simulink model "part4model"  (R2019b)
settings: Solver=VariableStepAuto  StartTime=0.0  StopTime=10.0  RelTol=1e-3
values from neighbouring files (symbols this model uses):
  encGain = (2*pi)/4096    (= 0.00153398078789)    [DC_Motor_Analysis.m]    (also in Part2.m; Part3.m; lqrPoles.mat; robust.mat)
  K_lqr = K_tilde(1:2)    [DC_Motor_Analysis.m]    (also in Part4.m = K(1:2); lqrPoles.mat = [-0.852723665026 -39.4121845033])
  ka = K(end)    [Part3.m]    (also in Part4.m; lqrPoles.mat = 316.227766017)
settings Model: Creator=justinf  LastModifiedBy=justinf

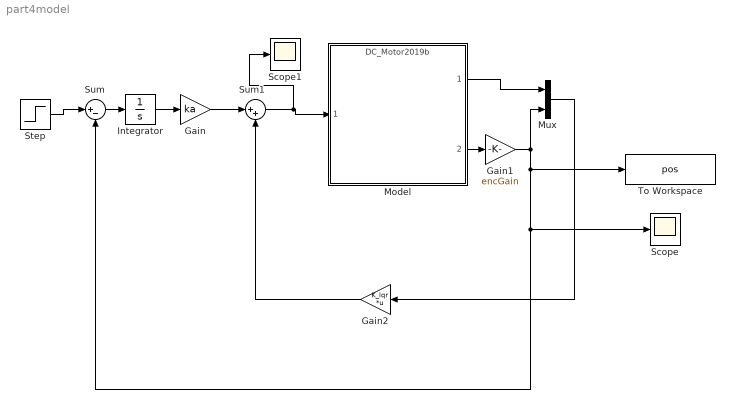
== system part4model ==
  Gain : Gain  Gain=ka
  Gain1 : Gain  Gain=encGain
  Gain2 : Gain  Gain=K_lqr  Multiplication=Matrix(K*u)
  Integrator : Integrator
  Model : ModelReference  ModelNameDialog=DC_Motor2019b.slxp  ModelReferenceVersion=1.20  CopyOfModelProtected=on
  Mux : Mux  Inputs=2
  Scope : Scope
  Scope1 : Scope
  Step : Step  Time=0  SampleTime=0
  Sum : Sum  Inputs=|+-
  Sum1 : Sum  Inputs=|++
  To Workspace : ToWorkspace  VariableName=pos  SampleTime=-1
  wires:
  Step/1 -> Sum/1
  Sum1/1 -> Scope1/1, Model/1
  Integrator/1 -> Gain/1
  Gain/1 -> Sum1/1
  Sum/1 -> Integrator/1
  Model/2 -> Gain1/1
  Gain1/1 -> Mux/2, To Workspace/1, Scope/1, Sum/2
  Mux/1 -> Gain2/1
  Gain2/1 -> Sum1/2
  Model/1 -> Mux/1
